simulink model "untitled"  (R2022a)
settings: Solver=ode4  StartTime=0.0  StopTime=4.9  FixedStep=0.01  RelTol=1e-3
undefined symbols (not defined in the file or in its folder): Discrete, Time
libraries: ctrlSharedLib x1
settings Model: Creator=20995  LastModifiedBy=20995

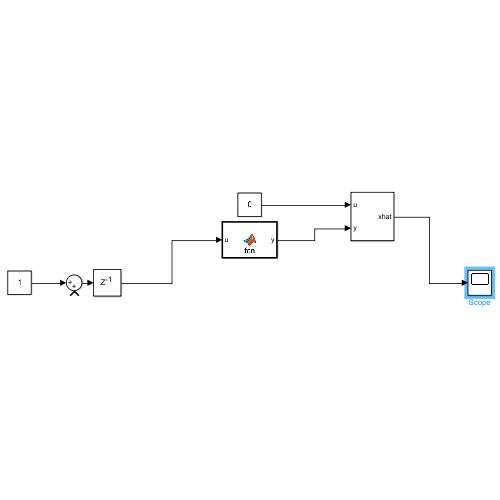
[thumbnail: Simulink's stored preview of the top-level diagram]
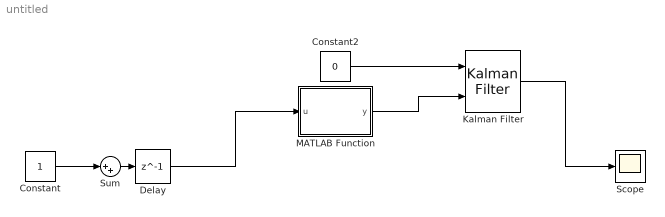
== system untitled ==
  Constant : Constant
  Constant2 : Constant  Value=0
  Delay : Delay  DelayLength=1
  Kalman Filter : ctrlSharedLib/Kalman Filter  TimeDomain=Discrete-Time  UseCurrentEstimator=on  ModelSource=Individual A, B, C, D matrices  ModelSourceVariable=ss(0.95,1,1,0,1)  A=1  B=1  C=1  D=0  NumberOfStates=1  NumberOfInputs=1  NumberOfOutputs=1  InitialEstimateSource=Dialog  X0=0  P0=10  UseK=off  UseGH=off  NumberOfProcessNoiseInputs=1  G=1  TimeInvariantG=on  H=0  TimeInvariantH=on  Q=0.001  TimeInvariantQ=on  R=10000  TimeInvariantR=on  N=0  TimeInvariantN=on  AddInputPort=on  AddEnablePort=off  OutputEstimatedY=off  OutputP=off  Ts=-1
  MATLAB Function : MATLAB Function  TreatAsAtomicUnit=on
  Scope : Scope
  Sum : Sum  Inputs=|++
  wires:
  Sum/1 -> Delay/1
  Constant/1 -> Sum/1
  Delay/1 -> MATLAB Function/1(u)
  Constant2/1 -> Kalman Filter/1
  Kalman Filter/1 -> Scope/1
  MATLAB Function/1(y) -> Kalman Filter/2

== matlab function untitled/MATLAB Function ==
  data: u input; y output
function y = fcn(u)
    data=load('C:\Users\20995\Desktop\homework_data_1.txt');
signal_values=data(:,2)
y = signal_values(u);
